simulink model "pd2"  (R2016b)
settings: Solver=VariableStepAuto  StartTime=0.0  StopTime=10.0  RelTol=1e-3
values from neighbouring files (symbols this model uses):
  den = [1 0.1313 1.109]    [UpdatedSimulinkValues-2.m]    (also in UpdatedSimulinkValuesalex1.m; part2a.m)
  Kd = G    [UpdatedSimulinkValues-2.m]    (also in UpdatedSimulinkValuesalex1.m; part2a.m = 0.1)
  Kp = G    [UpdatedSimulinkValues-2.m]    (also in UpdatedSimulinkValuesalex1.m; part2a.m = 0.1)
  num = [0.26*1.109*180/pi()]    [UpdatedSimulinkValues-2.m]    (also in UpdatedSimulinkValuesalex1.m; part2a.m)
settings Model: Creator=Alex  LastModifiedBy=Alex

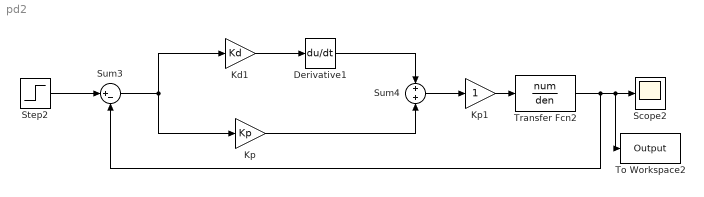
== system pd2 ==
  Derivative1 : Derivative
  Kd1 : Gain  Gain=Kd
  Kp : Gain  Gain=Kp
  Kp1 : Gain
  Scope2 : Scope
  Step2 : Step  SampleTime=0
  Sum3 : Sum  Inputs=|+-
  Sum4 : Sum
  To Workspace2 : ToWorkspace  VariableName=Output  SaveFormat=Timeseries  SampleTime=-1
  Transfer Fcn2 : TransferFcn  Numerator=num  Denominator=den
  wires:
  Step2/1 -> Sum3/1
  Transfer Fcn2/1 -> Sum3/2, To Workspace2/1, Scope2/1
  Sum4/1 -> Kp1/1
  Derivative1/1 -> Sum4/1
  Kd1/1 -> Derivative1/1
  Sum3/1 -> Kp/1, Kd1/1
  Kp/1 -> Sum4/2
  Kp1/1 -> Transfer Fcn2/1
